simulink model "Hall_sensor_120deg_2024a"  (R2024a)
settings: Solver=VariableStepAuto  StartTime=0.0  StopTime=1.5  MaxStep=1e-6  RelTol=1e-3
undefined symbols (not defined in the file): closed_loop, control_mode, D_duty_cycle, D_m, hall_errors, hall_errors_ON, I_duty_cycle, J_t, L_ss, lambda_m, P, P_duty_cycle, powergui, r_s, R_vs, sps_lib, T_m, tau_s, theta_v, V_bus
libraries: spsMosfetLib x6, spsSeriesRLCBranchLib x4, spsVoltageMeasurementLib x3, spsControlledCurrentSourceLib x3, slpidlib x2, eeGeneralControl x1, embmathops x1, spsPWMGeneratorDCDCLib x1, spsDCVoltageSourceLib x1
settings Model: SimulationMode=accelerator  Creator=baolo  LastModifiedBy=Aether
settings SolverCC: ZeroCrossAlgorithm=Adaptive
settings DebuggingCC: IgnoredZcDiagnostic=none

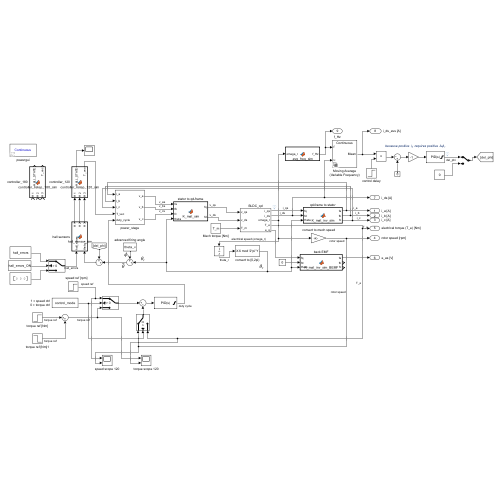
[thumbnail: Simulink's stored preview of the top-level diagram]
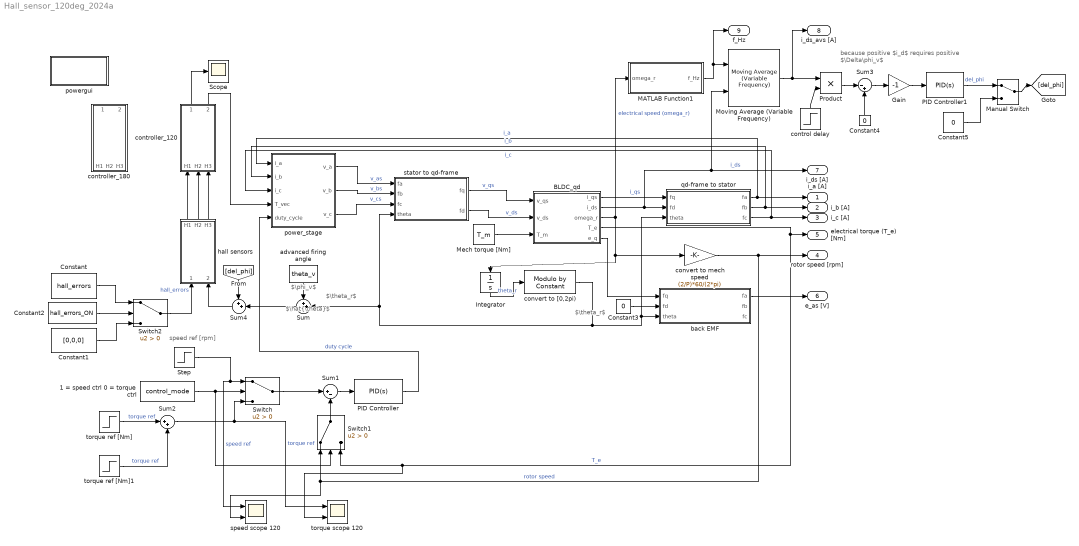
== system Hall_sensor_120deg_2024a ==
  note: because positive $i_d$ requires positive $\Delta\phi_v$
  note: $\phi_v$
  note: speed ref [rpm]
  note: $\theta_r$
  note: $\theta_r$
  note: $\hat{\theta}$
  1 = speed ctrl 0 = torque ctrl : Constant  Value=control_mode
  BLDC_qd : Subsystem
  Constant : Constant  Value=hall_errors
  Constant1 : Constant  Value=[0,0,0]
  Constant2 : Constant  Value=hall_errors_ON
  Constant3 : Constant  Value=0
  Constant4 : Constant  Value=0
  Constant5 : Constant  Value=0
  Gain : Gain  Gain=-1
  Integrator : Integrator
  MATLAB Function1 : MATLAB Function  TreatAsAtomicUnit=on
  Manual Switch : ManualSwitch
  Mech torque [Nm] : Constant  Value=T_m
  Moving Average (Variable Frequency) : eeGeneralControl/Moving Average (Variable Frequency)  VariantControl=Variant1  LabelModeActiveChoice=Continuous  f0=60  fmin=1  x0=0  BufferSize=32768  Ts=0
      settings: LibrarySourceBlock=|
      | ee_sl_lib/General Control/Moving Average
      | (Variable Frequency)
  PID Controller : slpidlib/PID Controller  Controller=PID  Form=Parallel  TimeDomain=Continuous-time  UseExternalTs=off  SampleTime=-1  IntegratorMethod=Forward Euler  FilterMethod=Forward Euler  ControllerParametersSource=internal  P=P_duty_cycle  I=I_duty_cycle  UseKiTs=off  D=D_duty_cycle  UseExternalDerivativeSource=off  N=100  UseFilter=on  TunerSelectOption=Transfer Function Based (PID Tuner App)  InitialConditionSource=internal  InitialConditionForIntegrator=0  InitialConditionForFilter=0  DifferentiatorICPrevScaledInput=0  ExternalReset=none  TrackingMode=off  Kt=1  LimitOutput=on  SatLimitsSource=internal  UpperSaturationLimit=1  LowerSaturationLimit=0  LinearizeAsGain=on  AntiWindupMode=none  Kb=1  LimitIntegrator=off  UpperIntegratorSaturationLimit=inf  LowerIntegratorSaturationLimit=-inf  POutMin=[]  POutMax=[]  IOutMin=[]  IOutMax=[]  DOutMin=[]  DOutMax=[]  NOutMin=[]  NOutMax=[]  SumOutMin=[]  SumOutMax=[]  SaturationOutMin=[]  SaturationOutMax=[]  PParamMin=[]  PParamMax=[]  IParamMin=[]  IParamMax=[]  DParamMin=[]  DParamMax=[]  NParamMin=[]  NParamMax=[]  KbParamMin=[]  KbParamMax=[]  KtParamMin=[]  KtParamMax=[]  KbOutMin=[]  KbOutMax=[]  KtOutMin=[]  KtOutMax=[]  IntegratorOutMin=[]  IntegratorOutMax=[]  FilterOutMin=[]  FilterOutMax=[]  SumI1OutMin=[]  SumI1OutMax=[]  SumI2OutMin=[]  SumI2OutMax=[]  SumI3OutMin=[]  SumI3OutMax=[]  SumI4OutMin=[]  SumI4OutMax=[]  SumDOutMin=[]  SumDOutMax=[]  DifferentiatorOutMin=[]  DifferentiatorOutMax=[]  FilterDiffOutCoefMin=[]  FilterDiffOutCoefMax=[]  ReciprocalOutMin=[]  ReciprocalOutMax=[]  SumDenOutMin=[]  SumDenOutMax=[]  SumNumOutMin=[]  SumNumOutMax=[]  DivideOutMin=[]  DivideOutMax=[]  UdiffTsProdOutMin=[]  UdiffTsProdOutMax=[]  NTsProdOutMin=[]  NTsProdOutMax=[]  UintegralTsProdOutMin=[]  UintegralTsProdOutMax=[]  UngainTsProdOutMin=[]  UngainTsProdOutMax=[]  ClampingZeroOutDataTypeStr=Inherit: Inherit via back propagation  ClampingZeroOutMin=[]  ClampingZeroOutMax=[]  FilterDenConstantOutDataTypeStr=Inherit: Inherit via back propagation  FilterDenConstantOutMin=[]  FilterDenConstantOutMax=[]  PCopyOutDataTypeStr=Inherit: Inherit via back propagation  PCopyOutMin=[]  PCopyOutMax=[]  NCopyOutDataTypeStr=Inherit: Inherit via back propagation  NCopyOutMin=[]  NCopyOutMax=[]  IntegratorContinuousStateAttributes=''  IntegratorStateMustResolveToSignalObject=off  IntegratorRTWStateStorageClass=Auto  FilterContinuousStateAttributes=''  FilterStateMustResolveToSignalObject=off  FilterRTWStateStorageClass=Auto  ParallelPVariant=InternalParameters  IdealPVariant=Disabled  IVariant=InternalParameters  DVariant=InternalParameters  IntegratorVariant=Continuous  SatVariant=Enabled  AWVariant=Passthrough  PCopyVariant=Disabled  TRVariant=Disabled  FdbkBlocksVariant=Forward  IdealPFdbkVariant=Disabled  SatFdbkVariant=Disabled  DerivativeFilterVariant=ContFilter  NVariant=InternalParameters  NCopyVariant=Disabled  FilterICVariant=InternalICsFilter  IntegratorICVariant=InternalICs  ExternalResetVariant=Disabled  TRSumVariant=Passthrough  SumFdbkVariant=Disabled  SumVariant=Sum_PID  TsampFilterVariant=InternalTs  TsampNgainVariant=Passthrough  TsampIntegralVariant=Disabled_SignalSpec  ExternalSaturationOutDataTypeStr=Inherit: Same as second input  DerivativeSourceVariant=ErrorSignal
  PID Controller1 : slpidlib/PID Controller  Controller=PID  Form=Parallel  TimeDomain=Continuous-time  UseExternalTs=off  SampleTime=-1  IntegratorMethod=Forward Euler  FilterMethod=Forward Euler  ControllerParametersSource=internal  P=0.136  I=4.464  UseKiTs=off  D=0  UseExternalDerivativeSource=off  N=100  UseFilter=on  TunerSelectOption=Transfer Function Based (PID Tuner App)  InitialConditionSource=internal  InitialConditionForIntegrator=0  InitialConditionForFilter=0  DifferentiatorICPrevScaledInput=0  ExternalReset=none  TrackingMode=off  Kt=1  LimitOutput=on  SatLimitsSource=internal  UpperSaturationLimit=pi/3  LowerSaturationLimit=-pi/3  LinearizeAsGain=on  AntiWindupMode=none  Kb=1  LimitIntegrator=off  UpperIntegratorSaturationLimit=inf  LowerIntegratorSaturationLimit=-inf  POutMin=[]  POutMax=[]  IOutMin=[]  IOutMax=[]  DOutMin=[]  DOutMax=[]  NOutMin=[]  NOutMax=[]  SumOutMin=[]  SumOutMax=[]  SaturationOutMin=[]  SaturationOutMax=[]  PParamMin=[]  PParamMax=[]  IParamMin=[]  IParamMax=[]  DParamMin=[]  DParamMax=[]  NParamMin=[]  NParamMax=[]  KbParamMin=[]  KbParamMax=[]  KtParamMin=[]  KtParamMax=[]  KbOutMin=[]  KbOutMax=[]  KtOutMin=[]  KtOutMax=[]  IntegratorOutMin=[]  IntegratorOutMax=[]  FilterOutMin=[]  FilterOutMax=[]  SumI1OutMin=[]  SumI1OutMax=[]  SumI2OutMin=[]  SumI2OutMax=[]  SumI3OutMin=[]  SumI3OutMax=[]  SumI4OutMin=[]  SumI4OutMax=[]  SumDOutMin=[]  SumDOutMax=[]  DifferentiatorOutMin=[]  DifferentiatorOutMax=[]  FilterDiffOutCoefMin=[]  FilterDiffOutCoefMax=[]  ReciprocalOutMin=[]  ReciprocalOutMax=[]  SumDenOutMin=[]  SumDenOutMax=[]  SumNumOutMin=[]  SumNumOutMax=[]  DivideOutMin=[]  DivideOutMax=[]  UdiffTsProdOutMin=[]  UdiffTsProdOutMax=[]  NTsProdOutMin=[]  NTsProdOutMax=[]  UintegralTsProdOutMin=[]  UintegralTsProdOutMax=[]  UngainTsProdOutMin=[]  UngainTsProdOutMax=[]  ClampingZeroOutDataTypeStr=Inherit: Inherit via back propagation  ClampingZeroOutMin=[]  ClampingZeroOutMax=[]  FilterDenConstantOutDataTypeStr=Inherit: Inherit via back propagation  FilterDenConstantOutMin=[]  FilterDenConstantOutMax=[]  PCopyOutDataTypeStr=Inherit: Inherit via back propagation  PCopyOutMin=[]  PCopyOutMax=[]  NCopyOutDataTypeStr=Inherit: Inherit via back propagation  NCopyOutMin=[]  NCopyOutMax=[]  IntegratorContinuousStateAttributes=''  IntegratorStateMustResolveToSignalObject=off  IntegratorRTWStateStorageClass=Auto  FilterContinuousStateAttributes=''  FilterStateMustResolveToSignalObject=off  FilterRTWStateStorageClass=Auto  ParallelPVariant=InternalParameters  IdealPVariant=Disabled  IVariant=InternalParameters  DVariant=InternalParameters  IntegratorVariant=Continuous  SatVariant=Enabled  AWVariant=Passthrough  PCopyVariant=Disabled  TRVariant=Disabled  FdbkBlocksVariant=Forward  IdealPFdbkVariant=Disabled  SatFdbkVariant=Disabled  DerivativeFilterVariant=ContFilter  NVariant=InternalParameters  NCopyVariant=Disabled  FilterICVariant=InternalICsFilter  IntegratorICVariant=InternalICs  ExternalResetVariant=Disabled  TRSumVariant=Passthrough  SumFdbkVariant=Disabled  SumVariant=Sum_PID  TsampFilterVariant=InternalTs  TsampNgainVariant=Passthrough  TsampIntegralVariant=Disabled_SignalSpec  ExternalSaturationOutDataTypeStr=Inherit: Same as second input  DerivativeSourceVariant=ErrorSignal
  Product : Product
  Scope : Scope
  Step : Step  Time=0.1  After=1000  SampleTime=0
  Sum : Sum  Inputs=++|
  Sum1 : Sum  Inputs=|+-
  Sum2 : Sum  Inputs=|++
  Sum3 : Sum  Inputs=|-+
  Sum4 : Sum  Inputs=++|
  Switch : Switch  Criteria=u2 > Threshold  SaturateOnIntegerOverflow=off  InputSameDT=off
  Switch1 : Switch  Criteria=u2 > Threshold  SaturateOnIntegerOverflow=off  InputSameDT=off
  Switch2 : Switch  Criteria=u2 > Threshold  SaturateOnIntegerOverflow=off  InputSameDT=off
  advanced firing angle : Constant  Value=theta_v
  back EMF : MATLAB Function  TreatAsAtomicUnit=on
  control delay : Step  Time=0.5  SampleTime=0
  controller_120 : MATLAB Function  TreatAsAtomicUnit=on
  controller_180 : MATLAB Function  TreatAsAtomicUnit=on
  convert to [0,2pi) : embmathops/Modulo by Constant  Denominator=2*pi  SimulateUsing=Code generation
      settings: LibrarySourceBlock=embeddedMathLib/Modulo by Constant
  convert to mech speed : Gain  Gain=(2/P)*60/(2*pi)
  hall sensors : MATLAB Function  TreatAsAtomicUnit=on
  power_stage : Subsystem
  powergui : Subsystem  Priority=1  AncestorBlock=sps_lib/powergui  InitFcn=powergui( 'InitFcn_Callback' , gcb , 0 , [ ] );  mask(PSB option menu block){SimulationMode=Continuous, SampleTime=50e-6, frequency=60, Iterations=50, frequencyindice=0, Pbase=100e6, ErrMax=1e-4, UnitsV=kV, UnitsW=MW, buscounter=0, FunctionMessages=off, echomessages=off, EnableUseOfTLC=off, CurrentSourceSwitches=off, DisableSnubberDevices=off, DisableRonSwitches=off, DisableVfSwitches=off, DisplayEquations=off, AutomaticDiscreteSolvers=off, SolverType=Tustin/Backward Euler (TBE), Interpol=off, ExternalGateDelay=off, methode=off, Ts=100, x0status=blocks, SPID=on, SwTol=0, HookPort=off, NonlinearTolerance=1e-4, nMaxIteration=100, ContinueOnMaxIteration=off, RestoreLinks=warning, ResistiveCurrentMeasurement=off, Frange=[0:2:500], Ylog=off, Xlog=on, ShowGrid=off, save=off, variable=ZData, structure=0, ZoomFFT=off, StartTime=0.0, cycles=1, DisplayStyle=1, fundamental=60, FreqAxis=off, MaxFrequency=1000, frequencyindicesteady=1, RmsSteady=1, display=off}
      mask prompts: SimulationMode "Simulation type:"; SampleTime "Sample time (s):"; frequency "Frequency (Hz):"; Iterations "Max iterations"; frequencyindice "Frequency (Hz)"; Pbase "Base power (VA)"; ErrMax "PQ tolerance (pu)"; UnitsV "Voltage units"; UnitsW "Power units"; buscounter "Load flow bus counter"; FunctionMessages "Disable Specialized Power Systems warnings"; echomessages "Display Specialized Power Systems compilation messages"; EnableUseOfTLC "Use TLC file when in Accelerator Simulation Mode and for code generation"; CurrentSourceSwitches "Disable ideal switching"; DisableSnubberDevices "Disable snubbers in switching devices"; DisableRonSwitches "Disable Ron resistances in switching devices"; DisableVfSwitches "Disable forward voltages in switching devices"; DisplayEquations "Display circuit differential equations"; AutomaticDiscreteSolvers "Automatically handle Discrete solver and Advanced tab solver settings of blocks"; SolverType "Discrete solver"; Interpol "Interpolate switching events"; ExternalGateDelay "Use time-stamped gate signals"; methode "Store switching topologies"; Ts "Buffer size (MBytes):"; x0status "Start simulation with initial electrical states from:"; SPID "Use ideal switching devices"; SwTol "Switch tolerance"; HookPort "Allow multiple powergui blocks"; NonlinearTolerance "Solver tolerance"; nMaxIteration "Maximum number of iterations"; ContinueOnMaxIteration "Continue Simulation if maximum number of iterations is reached"; RestoreLinks "Restore disabled links of Simscape Power Systems ST blocks:"; ResistiveCurrentMeasurement "Use non ideal current measurement blocks (1e-4Ohm internal resistance)"; Frange "Frequency Range"; Ylog "Log impedance"; Xlog "log Frequency"; ShowGrid "grid"; save "Save Data To Workspace"; variable "Variable Name"; structure "Structure Name (PSBFFTSCOPE)"; ZoomFFT "ZoomFFT (PSBFFTSCOPE)"; StartTime "Start Time (PSBFFTSCOPE)"; cycles "Cycles (PSBFFTSCOPE)"; DisplayStyle "Display style (PSBFFTSCOPE)"; fundamental "Fundamental (PSBFFTSCOPE)"; FreqAxis "Frequency Axis (PSBFFTSCOPE)"; MaxFrequency "Max Frequency (PSBFFTSCOPE)"; frequencyindicesteady "Frequency indice (STEADYSTATE)"; RmsSteady "RMS display (STEADYSTATE)"; display "Display Results"
      mask help: Set simulation type, simulation parameters, and preferences.
      mask init:
      | dispMessage = '';
      | dispMessage = powergui('MaskInitialization',gcb,SimulationMode,SampleTime);
      settings: LibrarySourceBlock=sps_lib/powergui  PreSaveFcn=powergui( 'PreSaveFcn_Callback' , gcb , [ ] , [ ] );  OpenFcn=sps_rtmsupport('OpenFcn',gcbh)
      mask Help: helpview(psbhelp)
      mask TypeOptions SimulationMode: Continuous | Discrete | Phasor | Discrete phasor
      mask Callback SimulationMode: powergui('SimulationType',[],[],gcb);
      mask TypeOptions UnitsV: V | kV
      mask TypeOptions UnitsW: W | kW | MW
      mask Callback CurrentSourceSwitches: powergui('SimulationType',[],[],gcb);
      mask Callback AutomaticDiscreteSolvers: powergui('SimulationType',[],[],gcb);
      mask TypeOptions SolverType: Tustin/Backward Euler (TBE) | Tustin | Backward Euler
      mask Callback SolverType: powergui('SimulationType',[],[],gcb);
      mask Callback Interpol: powergui('SimulationType',[],[],gcb);
      mask Callback ExternalGateDelay: powergui('SimulationType',[],[],gcb);
      mask Callback methode: powergui('SimulationType',[],[],gcb);
      mask TypeOptions x0status: blocks | steady | zero
      mask TypeOptions RestoreLinks: yes | warning | no
      mask Callback display: sps_rtmsupport('parametereditingmodes',gcbh) % Will be executed last in parameter callbacks to ensure mask enable consistency
      mask DialogControl SolverTab Prompt: Solver
      mask DialogControl AutoSolverNote Prompt: The Simulation type parameter is governed by Simulink. To access the Powergui solver settings, unselect auto (Automatic solver selection) solver in the Simulink solver options.
      mask DialogControl Apps Prompt: Apps
      mask DialogControl StateAnalyzer Prompt: Measurements and States Analyzer
      mask DialogControl StateAnalyzer Callback: powerStates(bdroot(gcb))
      mask DialogControl LineParameterCalculator Prompt: Line Parameter Calculator
      mask DialogControl LineParameterCalculator Callback:
      | close_system(gcb)
      | powerLineParameters
      mask DialogControl CableParameterCalculator Prompt: Cable Parameter Calculator
      mask DialogControl CableParameterCalculator Callback:
      | close_system(gcb)
      | powerCableParameters
      mask DialogControl LineDecoupler Prompt: Line Decoupler
      mask DialogControl LineDecoupler Tooltip: Click to replace selected Distributed Parameters Line blocks with Decoupling Line blocks
      mask DialogControl LineDecoupler Callback:
      | close_system(gcb);
      | DecouplingLineReplace(gcs)
      mask DialogControl LoadFlowAnalyzer Prompt: Load Flow Analyzer
      mask DialogControl LoadFlowAnalyzer Callback:
      | close_system(gcb)
      | powerLoadFlow
      mask DialogControl LoadFlowParameters Prompt: Load Flow Parameters
      mask DialogControl ImpedanceCalculator Prompt: Impedance Calculator
      mask DialogControl ImpedanceCalculator Callback:
      | close_system(gcb);
      | powerImpedance(bdroot(gcs));
      mask DialogControl FFTAnalyzer Prompt: FFT Analyzer
      mask DialogControl FFTAnalyzer Callback:
      | close_system(gcb)
      | power_fftscope(bdroot(gcb),gcb)
      mask DialogControl LinearSystemAnalyzer Prompt: Linear System Analyzer
      mask DialogControl LinearSystemAnalyzer Callback:
      | close_system(gcb)
      | power_ltiview(bdroot(gcb))
      mask DialogControl HysteresisDesigner Prompt: Hysteresis Designer
      mask DialogControl HysteresisDesigner Callback:
      | close_system(gcb)
      | powerHysteresis('hysteresis.mat')
      mask DialogControl BlockCustomizer Prompt: Block Customizer
      mask DialogControl BlockCustomizer Callback:
      | close_system(gcb);
      | power_customize;
      mask DialogControl ReportGenerator Prompt: Report Generator
      mask DialogControl ReportGenerator Callback:
      | close_system(gcb)
      | power_report(bdroot(gcb))
      mask DialogControl obsolete Prompt: ...
      mask DialogControl MachineInitialization Prompt: Machine Initialization
      mask DialogControl MachineInitialization Callback:
      | close_system(gcb)
      | powericon('machineInitTool',bdroot(gcb),gcb)
      mask DialogControl Preferences Prompt: Preferences
      mask DialogControl Solver Prompt: Solver
      mask DialogControl SolverDetails Prompt: Solver details for nonlinear elements
      mask Display: color('blue'),disp(dispMessage)
  qd-frame to stator : MATLAB Function  TreatAsAtomicUnit=on
  speed scope 120 : Scope  NumInputPorts=2
  stator to qd-frame : MATLAB Function  TreatAsAtomicUnit=on
  torque ref [Nm] : Step  Time=0.1  After=1e-1  SampleTime=0  ZeroCross=off
  torque ref [Nm]1 : Step  After=-0.5e-1  SampleTime=0
  torque scope 120 : Scope  NumInputPorts=2
  i_a [A] : Outport
  i_b [A] : Outport  Port=2
  i_c [A] : Outport  Port=3
  rotor speed [rpm] : Outport  Port=4
  electrical torque (T_e) [Nm] : Outport  Port=5
  e_as [V] : Outport  Port=6
  i_ds [A] : Outport  Port=7
  i_ds_avs [A] : Outport  Port=8
  f_Hz : Outport  Port=9
  wires:
  stator to qd-frame/1(fq) -> BLDC_qd/1(v_qs)  "v_qs"
  stator to qd-frame/2(fd) -> BLDC_qd/2(v_ds)  "v_ds"
  Mech torque [Nm]/1 -> BLDC_qd/3(T_m)
  BLDC_qd/1(i_qs) -> qd-frame to stator/1(fq)  "i_qs"
  BLDC_qd/2(i_ds) -> i_ds [A]/1, Moving Average (Variable Frequency)/2, qd-frame to stator/2(fd)  "i_ds"
  BLDC_qd/3(omega_r) -> MATLAB Function1/1(omega_r), convert to mech speed/1, Integrator/1  "electrical speed (omega_r)"
  convert to [0,2pi)/1 -> stator to qd-frame/4(theta), Sum/2, back EMF/3(theta), qd-frame to stator/3(theta)
  power_stage/1(v_a) -> stator to qd-frame/1(fa)  "v_as"
  power_stage/2(v_b) -> stator to qd-frame/2(fb)  "v_bs"
  power_stage/3(v_c) -> stator to qd-frame/3(fc)  "v_cs"
  Integrator/1 -> convert to [0,2pi)/1  "theta_r"
  hall sensors/1(H1) -> controller_120/1(H1)
  hall sensors/2(H2) -> controller_120/2(H2)
  hall sensors/3(H3) -> controller_120/3(H3)
  advanced firing angle/1 -> Sum/1
  Sum/1 -> Sum4/2
  qd-frame to stator/1(fa) -> power_stage/1(i_a), i_a [A]/1  "i_a"
  qd-frame to stator/2(fb) -> power_stage/2(i_b), i_b [A]/1  "i_b"
  qd-frame to stator/3(fc) -> power_stage/3(i_c), i_c [A]/1  "i_c"
  convert to mech speed/1 -> rotor speed [rpm]/1, speed scope 120/2, Switch1/1  "rotor speed"
  BLDC_qd/4(T_e) -> torque scope 120/2, Switch1/3, electrical torque (T_e) [Nm]/1  "T_e"
  1 = speed ctrl 0 = torque ctrl/1 -> Switch/2, Switch1/2
  Step/1 -> speed scope 120/1, Switch/1  "speed ref"
  Sum2/1 -> torque scope 120/1, Switch/3  "torque ref"
  Switch1/1 -> Sum1/2
  Switch/1 -> Sum1/1
  Sum1/1 -> PID Controller/1
  PID Controller/1 -> power_stage/5(duty_cycle)  "duty cycle"
  torque ref [Nm]/1 -> Sum2/1  "torque ref"
  torque ref [Nm]1/1 -> Sum2/2  "torque ref"
  Constant/1 -> Switch2/1
  Switch2/1 -> hall sensors/1(hall_errors)  "hall_errors"
  Constant1/1 -> Switch2/3
  controller_120/2(T_vec) -> power_stage/4(T_vec)
  controller_120/1(HALL_STATE) -> Scope/1
  Constant2/1 -> Switch2/2
  BLDC_qd/5(e_q) -> back EMF/1(fq)
  Constant3/1 -> back EMF/2(fd)
  back EMF/1(fa) -> e_as [V]/1
  Moving Average (Variable Frequency)/1 -> Product/1, i_ds_avs [A]/1
  MATLAB Function1/1(f_Hz) -> f_Hz/1, Moving Average (Variable Frequency)/1
  Constant4/1 -> Sum3/2
  Sum3/1 -> Gain/1
  PID Controller1/1 -> Manual Switch/1  "del_phi"
  [del_phi] -> Sum4/1
  Sum4/1 -> hall sensors/2(theta_r)
  Constant5/1 -> Manual Switch/2
  control delay/1 -> Product/2
  Product/1 -> Sum3/1
  Manual Switch/1 -> [del_phi]
  Gain/1 -> PID Controller1/1

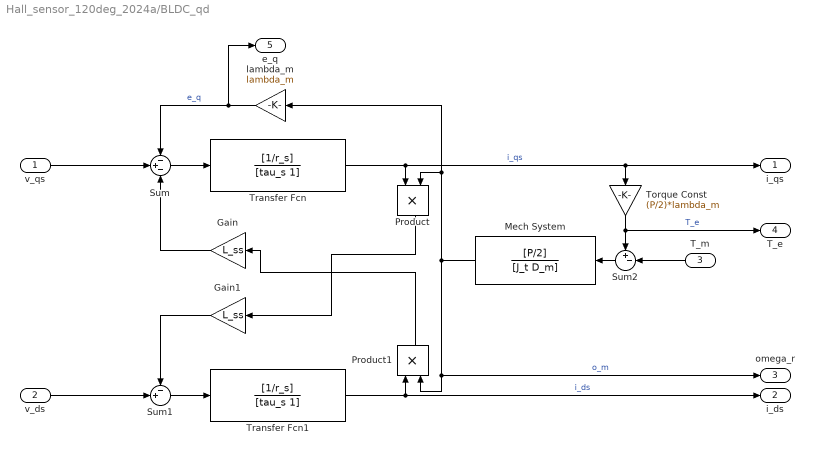
== system Hall_sensor_120deg_2024a/BLDC_qd ==
  v_qs : Inport
  v_ds : Inport  Port=2
  T_m : Inport  Port=3
  Gain : Gain  Gain=L_ss
  Gain1 : Gain  Gain=L_ss
  Mech System : TransferFcn  Numerator=[P/2]  Denominator=[J_t D_m]
  Product : Product
  Product1 : Product
  Sum : Sum  Inputs=-+-
  Sum1 : Sum  Inputs=-+|
  Sum2 : Sum  Inputs=+-|
  Torque Const : Gain  Gain=(P/2)*lambda_m
  Transfer Fcn : TransferFcn  Numerator=[1/r_s]  Denominator=[tau_s 1]
  Transfer Fcn1 : TransferFcn  Numerator=[1/r_s]  Denominator=[tau_s 1]
  lambda_m : Gain  Gain=lambda_m
  i_qs : Outport
  i_ds : Outport  Port=2
  omega_r : Outport  Port=3
  T_e : Outport  Port=4
  e_q : Outport  Port=5
  wires:
  T_m/1 -> Sum2/2
  Sum1/1 -> Transfer Fcn1/1
  Gain1/1 -> Sum1/1
  Product1/1 -> Gain/1
  Transfer Fcn1/1 -> i_ds/1, Product1/1  "i_ds"
  Mech System/1 -> lambda_m/1, Product/2, omega_r/1, Product1/2  "o_m"
  Torque Const/1 -> T_e/1, Sum2/1  "T_e"
  v_ds/1 -> Sum1/2
  Transfer Fcn/1 -> i_qs/1, Torque Const/1, Product/1  "i_qs"
  Product/1 -> Gain1/1
  Gain/1 -> Sum/3
  v_qs/1 -> Sum/2
  Sum/1 -> Transfer Fcn/1
  Sum2/1 -> Mech System/1
  lambda_m/1 -> e_q/1, Sum/1  "e_q"

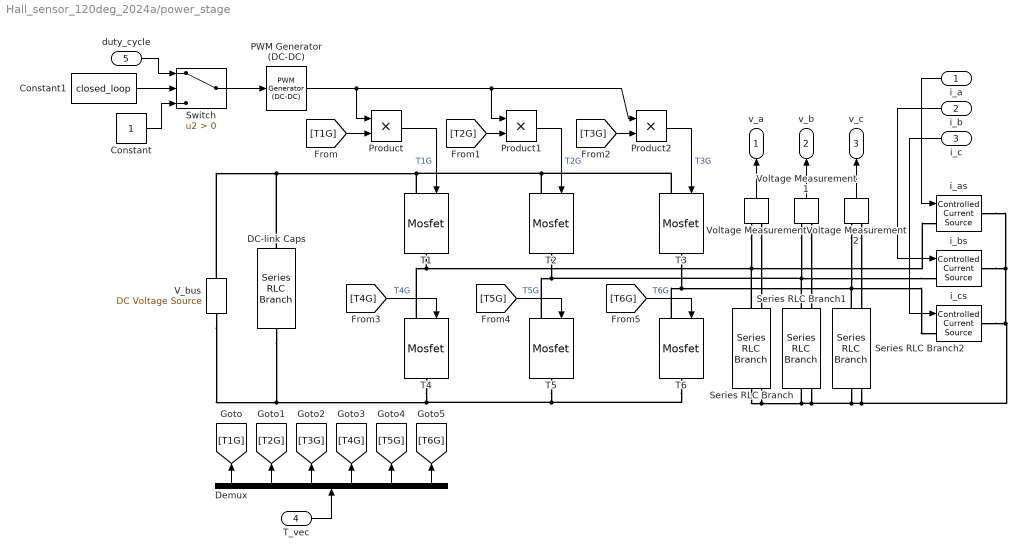
== system Hall_sensor_120deg_2024a/power_stage ==
  i_a : Inport
  i_b : Inport  Port=2
  i_c : Inport  Port=3
  T_vec : Inport  Port=4
  duty_cycle : Inport  Port=5
  Constant : Constant
  Constant1 : Constant  Value=closed_loop
  DC-link Caps : spsSeriesRLCBranchLib/Series RLC Branch  LConnTagsString=__new0  RConnTagsString=__new0  BranchType=RC  Resistance=1e-6  Inductance=0  SetiL0=off  InitialCurrent=0  Capacitance=100e-6  Setx0=off  InitialVoltage=0  Measurements=None
  Demux : Demux  Outputs=6
  PWM Generator (DC-DC) : spsPWMGeneratorDCDCLib/PWM Generator (DC-DC)  Fsw=f_SW_Hz  Ts=0
  Product : Product
  Product1 : Product
  Product2 : Product
  Series RLC Branch : spsSeriesRLCBranchLib/Series RLC Branch  LConnTagsString=__new0  RConnTagsString=__new0  BranchType=R  Resistance=R_vs  Inductance=0  SetiL0=off  InitialCurrent=0  Capacitance=inf  Setx0=off  InitialVoltage=0  Measurements=None
  Series RLC Branch1 : spsSeriesRLCBranchLib/Series RLC Branch  LConnTagsString=__new0  RConnTagsString=__new0  BranchType=R  Resistance=R_vs  Inductance=0  SetiL0=off  InitialCurrent=0  Capacitance=inf  Setx0=off  InitialVoltage=0  Measurements=None
  Series RLC Branch2 : spsSeriesRLCBranchLib/Series RLC Branch  LConnTagsString=__new0  RConnTagsString=__new0  BranchType=R  Resistance=R_vs  Inductance=0  SetiL0=off  InitialCurrent=0  Capacitance=inf  Setx0=off  InitialVoltage=0  Measurements=None
  Switch : Switch  Criteria=u2 > Threshold  SaturateOnIntegerOverflow=off  InputSameDT=off
  T{1..6} (6 alike) : spsMosfetLib/Mosfet  Ron=R_dsON_Ohm  Lon=0  Rd=0.01  Vfd=0.7  IC=0  Rs=1e5  Cs=inf  Measurements=off
  V_bus : spsDCVoltageSourceLib/DC Voltage Source  Amplitude=V_bus  Measurements=None
  Voltage Measurement : spsVoltageMeasurementLib/Voltage Measurement  PhasorSimulation=off  OutputType=Complex  PSBequivalent=0
  Voltage Measurement1 : spsVoltageMeasurementLib/Voltage Measurement  PhasorSimulation=off  OutputType=Complex  PSBequivalent=0
  Voltage Measurement2 : spsVoltageMeasurementLib/Voltage Measurement  PhasorSimulation=off  OutputType=Complex  PSBequivalent=0
  i_as : spsControlledCurrentSourceLib/Controlled Current Source  Initialize=on  Source_Type=AC  Amplitude=0  Phase=0  Frequency=0  Measurements=None
  i_bs : spsControlledCurrentSourceLib/Controlled Current Source  Initialize=on  Source_Type=AC  Amplitude=0  Phase=0  Frequency=0  Measurements=None
  i_cs : spsControlledCurrentSourceLib/Controlled Current Source  Initialize=on  Source_Type=AC  Amplitude=0  Phase=0  Frequency=0  Measurements=None
  v_a : Outport
  v_b : Outport  Port=2
  v_c : Outport  Port=3
  wires:
  T_vec/1 -> Demux/1
  Product1/1 -> T2/1  "T2G"
  PWM Generator (DC-DC)/1 -> Product/1, Product2/1, Product1/1
  Demux/6 -> [T6G]
  [T4G] -> T4/1  "T4G"
  [T5G] -> T5/1  "T5G"
  Demux/4 -> [T4G]
  Voltage Measurement/1 -> v_a/1
  [T2G] -> Product1/2
  Voltage Measurement1/1 -> v_b/1
  Voltage Measurement2/1 -> v_c/1
  i_a/1 -> i_as/1
  Demux/1 -> [T1G]
  Demux/5 -> [T5G]
  [T6G] -> T6/1  "T6G"
  i_c/1 -> i_cs/1
  Product/1 -> T1/1  "T1G"
  [T3G] -> Product2/2
  i_b/1 -> i_bs/1
  Product2/1 -> T3/1  "T3G"
  Demux/2 -> [T2G]
  Demux/3 -> [T3G]
  [T1G] -> Product/2
  duty_cycle/1 -> Switch/1
  Constant/1 -> Switch/3
  Constant1/1 -> Switch/2
  Switch/1 -> PWM Generator (DC-DC)/1
  connections:
  i_bs/LConn1 -- Voltage Measurement1/LConn1 -- Series RLC Branch1/LConn1 -- T2/RConn1 -- T5/LConn1
  DC-link Caps/RConn1 -- V_bus/LConn1 -- T4/RConn1 -- T6/RConn1 -- T5/RConn1
  DC-link Caps/LConn1 -- V_bus/RConn1 -- T1/LConn1 -- T3/LConn1 -- T2/LConn1
  T4/LConn1 -- T1/RConn1 -- Voltage Measurement/LConn1 -- Series RLC Branch/LConn1 -- i_as/LConn1
  T3/RConn1 -- T6/LConn1 -- Voltage Measurement2/LConn1 -- Series RLC Branch2/LConn1 -- i_cs/LConn1
  Series RLC Branch/RConn1 -- Voltage Measurement/LConn2 -- i_bs/RConn1 -- i_as/RConn1 -- i_cs/RConn1 -- Voltage Measurement2/LConn2 -- Series RLC Branch2/RConn1 -- Voltage Measurement1/LConn2 -- Series RLC Branch1/RConn1

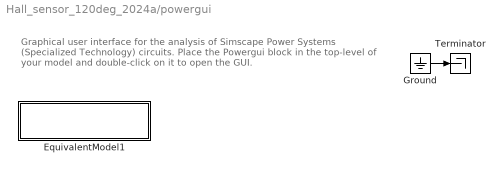
== system Hall_sensor_120deg_2024a/powergui ==
  note: Graphical user interface for the analysis of
      | Simscape Power Systems (Specialized Technology) circuits.
      | Place the Powergui block in the top-level of your model and double-click
      | on it to open the GUI.
  EquivalentModel1 : Subsystem  mask{SwTol=SwTol}
      mask prompts: SwTol "SwitchTolerance"
      mask init:
      | S  = GetDataForEquivalentModel('SPID',gcbh,SwTol);
      mask Display:
      | color('blue')
      | disp('EQUIVALENT CIRCUIT\nSPID')
  Ground : Ground
  Terminator : Terminator
  wires:
  Ground/1 -> Terminator/1

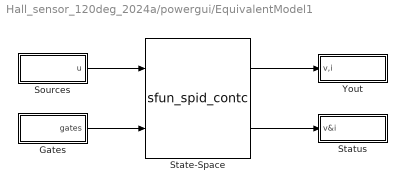
== system Hall_sensor_120deg_2024a/powergui/EquivalentModel1 ==
  Gates : Subsystem
  Sources : Subsystem
  State-Space : S-Function  FunctionName=sfun_spid_contc  Parameters=S.Mg, [S.nb.x S.nb.u S.nb.y S.nb.s], S.x0, S.MgColNames, S.SwitchVf, S.SwitchType, S.SwitchGateInitialValue, S.SwitchTolerance,S.SaveMatrices,S.BufferSize  SFunctionDeploymentMode=off  EnableBusSupport=off
  Status : Subsystem
  Yout : Subsystem
  wires:
  State-Space/1 -> Yout/1(v,i)
  State-Space/2 -> Status/1(v&i)
  Gates/1(gates) -> State-Space/2
  Sources/1(u) -> State-Space/1

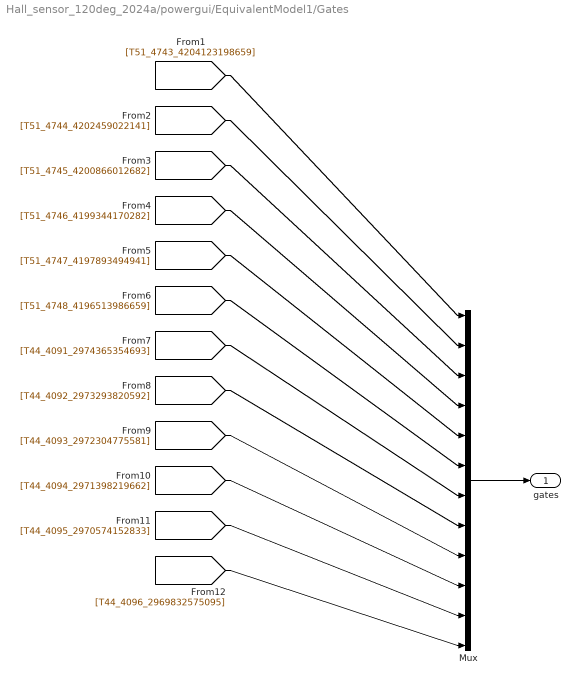
== system Hall_sensor_120deg_2024a/powergui/EquivalentModel1/Gates ==
  Mux : Mux  Inputs=[1 1 1 1 1 1 1 1 1 1 1 1]
  gates : Outport  VectorParamsAs1DForOutWhenUnconnected=off
  wires:
  Mux/1 -> gates/1
  [T51_4743_4204123198659] -> Mux/1
  [T51_4744_4202459022141] -> Mux/2
  [T51_4745_4200866012682] -> Mux/3
  [T51_4746_4199344170282] -> Mux/4
  [T51_4747_4197893494941] -> Mux/5
  [T51_4748_4196513986659] -> Mux/6
  [T44_4091_2974365354693] -> Mux/7
  [T44_4092_2973293820592] -> Mux/8
  [T44_4093_2972304775581] -> Mux/9
  [T44_4094_2971398219662] -> Mux/10
  [T44_4095_2970574152833] -> Mux/11
  [T44_4096_2969832575095] -> Mux/12

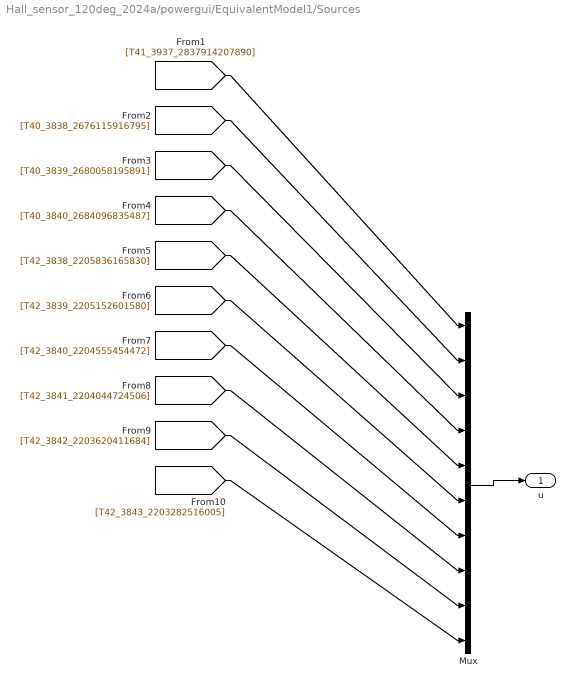
== system Hall_sensor_120deg_2024a/powergui/EquivalentModel1/Sources ==
  Mux : Mux  Inputs=[1 1 1 1 1 1 1 1 1 1]
  u : Outport  VectorParamsAs1DForOutWhenUnconnected=off
  wires:
  Mux/1 -> u/1
  [T41_3937_2837914207890] -> Mux/1
  [T40_3838_2676115916795] -> Mux/2
  [T40_3839_2680058195891] -> Mux/3
  [T40_3840_2684096835487] -> Mux/4
  [T42_3838_2205836165830] -> Mux/5
  [T42_3839_2205152601580] -> Mux/6
  [T42_3840_2204555454472] -> Mux/7
  [T42_3841_2204044724506] -> Mux/8
  [T42_3842_2203620411684] -> Mux/9
  [T42_3843_2203282516005] -> Mux/10

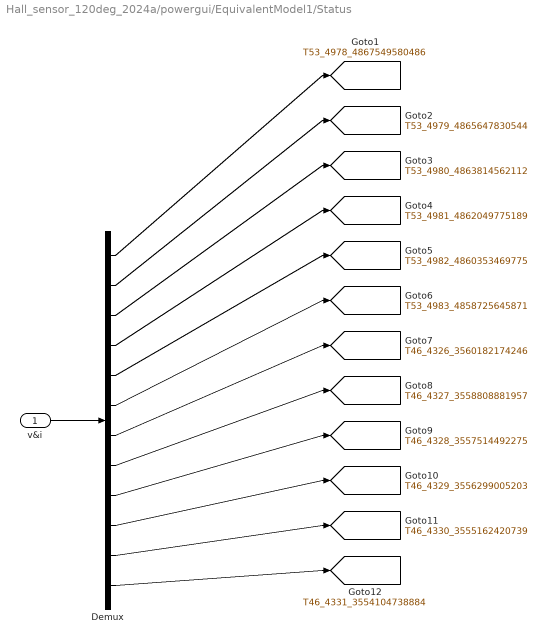
== system Hall_sensor_120deg_2024a/powergui/EquivalentModel1/Status ==
  v&i : Inport
  Demux : Demux  Outputs=[2 2 2 2 2 2 2 2 2 2 2 2]
  tag scope: T46_4326_3560182174246=global, T46_4327_3558808881957=global, T46_4328_3557514492275=global, T46_4329_3556299005203=global, T46_4330_3555162420739=global, T46_4331_3554104738884=global, T53_4978_4867549580486=global, T53_4979_4865647830544=global, T53_4980_4863814562112=global, T53_4981_4862049775189=global, T53_4982_4860353469775=global, T53_4983_4858725645871=global
  wires:
  v&i/1 -> Demux/1
  Demux/1 -> [T53_4978_4867549580486]
  Demux/2 -> [T53_4979_4865647830544]
  Demux/3 -> [T53_4980_4863814562112]
  Demux/4 -> [T53_4981_4862049775189]
  Demux/5 -> [T53_4982_4860353469775]
  Demux/6 -> [T53_4983_4858725645871]
  Demux/7 -> [T46_4326_3560182174246]
  Demux/8 -> [T46_4327_3558808881957]
  Demux/9 -> [T46_4328_3557514492275]
  Demux/10 -> [T46_4329_3556299005203]
  Demux/11 -> [T46_4330_3555162420739]
  Demux/12 -> [T46_4331_3554104738884]

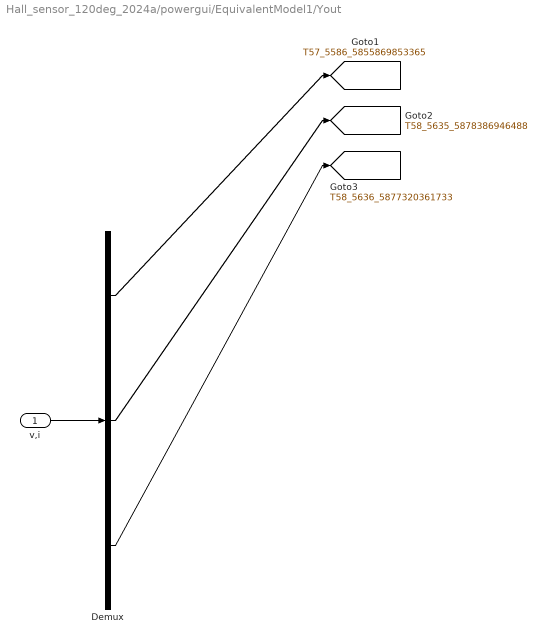
== system Hall_sensor_120deg_2024a/powergui/EquivalentModel1/Yout ==
  v,i : Inport
  Demux : Demux  Outputs=[1 1 1]
  tag scope: T57_5586_5855869853365=global, T58_5635_5878386946488=global, T58_5636_5877320361733=global
  wires:
  v,i/1 -> Demux/1
  Demux/1 -> [T57_5586_5855869853365]
  Demux/2 -> [T58_5635_5878386946488]
  Demux/3 -> [T58_5636_5877320361733]

== matlab function Hall_sensor_120deg_2024a/qd-frame to stator ==
  data: fa output; fb output; fc output; fq input; fd input; theta input
function [fa,fb,fc] = K_mat_inv_sim(fq,fd,theta)
[fa,fb,fc] = K_mat_inv(fq,fd,theta);

== matlab function Hall_sensor_120deg_2024a/stator to qd-frame ==
  data: fa input; fq output; fb input; fc input; theta input; fd output
function [fq,fd] = K_mat_sim(fa,fb,fc,theta)
[fq,fd] = K_mat(fa,fb,fc,theta);

== matlab function Hall_sensor_120deg_2024a/back EMF ==
  data: fa output; fb output; fc output; fq input; fd input; theta input
function [fa,fb,fc] = K_mat_inv_sim_BEMF(fq,fd,theta)
[fa,fb,fc] = K_mat_inv(fq,fd,theta);

== matlab function Hall_sensor_120deg_2024a/hall sensors ==
  data: hall_errors input; theta_r input; H1 output; H2 output; H3 output
function [H1,H2,H3] = hall_sensor_sim(hall_errors, theta_r)
[H1,H2,H3] = hall_sensor(theta_r, hall_errors);
end

== matlab function Hall_sensor_120deg_2024a/controller_120 ==
  data: H1 input; HALL_STATE output; H2 input; H3 input; T_vec output
function [HALL_STATE, T_vec] = controller_6step_120_sim(H1,H2,H3)
[HALL_STATE, T_vec] = controller_6step_120(H1,H2,H3);
end

== matlab function Hall_sensor_120deg_2024a/controller_180 ==
  data: H1 input; HALL_STATE output; H2 input; H3 input; T_vec output
function [HALL_STATE, T_vec] = controller_6step_180_sim(H1,H2,H3)
[HALL_STATE, T_vec] = controller_6step_180(H1,H2,H3);
end

== matlab function Hall_sensor_120deg_2024a/MATLAB Function1 ==
  data: omega_r input; f_Hz output
function f_Hz = avg_freq_sim(omega_r)
f_Hz = avg_freq(omega_r);
